simulink model "lateral_naolinear"  (R2021b)
settings: Solver=FixedStepAuto  StartTime=0.0  StopTime=2  FixedStep=1e-3  RelTol=1e-3
values from neighbouring files (symbols this model uses):
  y0 = y0s(i)    [avaliarLinearidadeLateral.m]
  yr = yrs(j)    [avaliarFollowline.m]
undefined symbols (not defined in the file or in its folder): Kpsi, Ky, psi0, psirMax, v
settings Model: Creator=mmaximo  LastModifiedBy=buga
settings SolverCC: AlgebraicLoopSolver=TrustRegion
settings DebuggingCC: SFMachineParentedDataDiag=warning

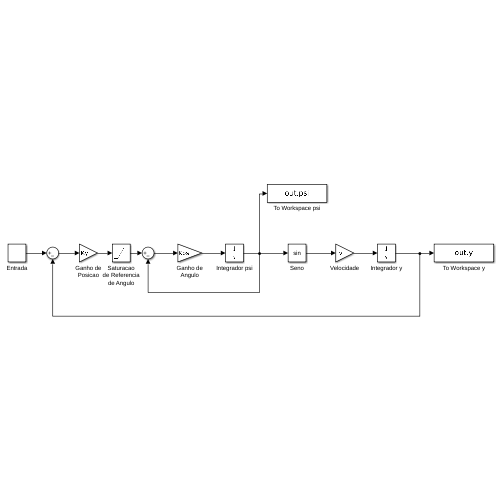
[thumbnail: Simulink's stored preview of the top-level diagram]
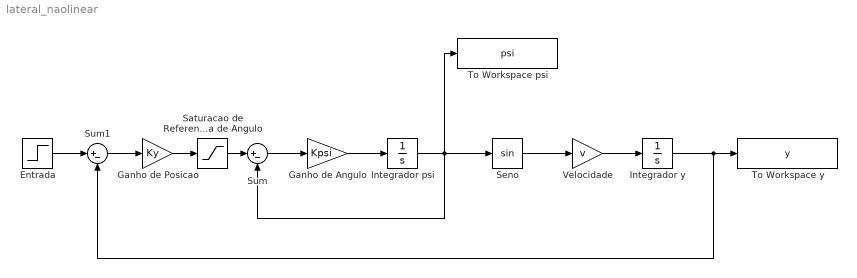
== system lateral_naolinear ==
  Entrada : Step  Time=0  After=yr  SampleTime=0
  Ganho de Angulo : Gain  Gain=Kpsi
  Ganho de Posicao : Gain  Gain=Ky
  Integrador psi : Integrator  InitialCondition=psi0
  Integrador y : Integrator  InitialCondition=y0
  Saturacao de Referencia de Angulo : Saturate  UpperLimit=psirMax  LowerLimit=-psirMax
  Seno : Trigonometry
  Sum : Sum  Inputs=|+-
  Sum1 : Sum  Inputs=|+-
  To Workspace psi : ToWorkspace  VariableName=psi  SaveFormat=Structure With Time  SampleTime=-1
  To Workspace y : ToWorkspace  VariableName=y  SaveFormat=Structure With Time  SampleTime=-1
  Velocidade : Gain  Gain=v
  wires:
  Entrada/1 -> Sum1/1
  Sum1/1 -> Ganho de Posicao/1
  Sum/1 -> Ganho de Angulo/1
  Ganho de Angulo/1 -> Integrador psi/1
  Seno/1 -> Velocidade/1
  Velocidade/1 -> Integrador y/1
  Integrador y/1 -> Sum1/2, To Workspace y/1
  Ganho de Posicao/1 -> Saturacao de Referencia de Angulo/1
  Saturacao de Referencia de Angulo/1 -> Sum/1
  Integrador psi/1 -> Sum/2, To Workspace psi/1, Seno/1
